simulink model "pll"  (Simulink 9.2)
settings: Solver=ode45  StartTime=0.0  StopTime=40  MaxStep=0.0001  RelTol=1e-3  EnableMultiTasking=on
libraries: simulink x2
settings Model: Creator=buddyugwumba1  LastModifiedBy=buddyugwumba1
settings OptimizationCC: InitFltsAndDblsToZero=on
settings DebuggingCC: SaveWithParameterizedLinksMsg=none  SignalResolutionControl=TryResolveAllWithWarning  SolverPrmCheckMsg=warning  MultiTaskDSMMsg=warning  MultiTaskCondExecSysMsg=none  FcnCallInpInsideContextMsg=error  StateNameClashWarn=none
settings SFSimCC: SimUseLocalCustomCode=on
settings RTWCC: RTWUseLocalCustomCode=on
settings GRTTargetCC: TargetFcnLib=ansi_tfl_tmw.mat  GeneratePreprocessorConditionals=Use local settings
settings ConfigComp: CovExternalEMLEnable=on

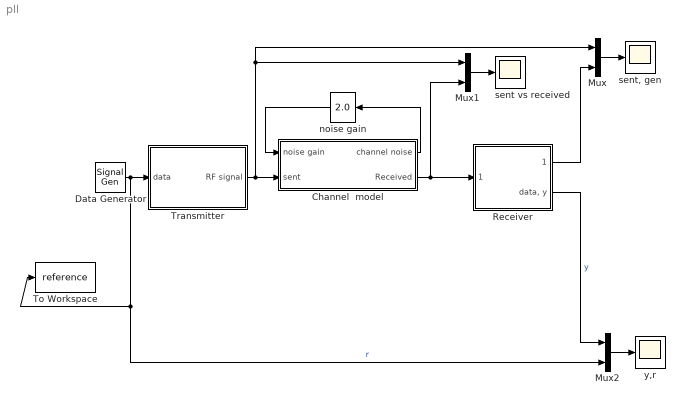
== system pll ==
  Channel  model : Subsystem
  Data Generator : SignalGenerator  WaveForm=square  Amplitude=2  Frequency=0.05
  Mux : Mux  Inputs=2
  Mux1 : Mux  Inputs=2
  Mux2 : Mux  Inputs=2
  Receiver : Subsystem
  To Workspace : ToWorkspace  VariableName=reference  SaveFormat=Structure With Time  SampleTime=-1
  Transmitter : Subsystem
  noise gain : simulink/Math Operations/Slider Gain  gain=2.0  low=0  high=2
  sent vs received : Scope
  "sent, gen" : Scope
  y,r : Scope
  wires:
  Mux/1 -> "sent, gen"/1
  Receiver/1(rep. sin) -> Mux/2
  Transmitter/1(RF signal) -> Channel  model/2(sent), Mux/1, Mux1/1
  Channel  model/2(Received) -> Receiver/1(rcvd. sig), Mux1/2
  Mux1/1 -> sent vs received/1
  Mux2/1 -> y,r/1
  Data Generator/1 -> To Workspace/1, Mux2/2, Transmitter/1(data)  "r"
  noise gain/1 -> Channel  model/1(noise gain)
  Channel  model/1(channel noise) -> noise gain/1
  Receiver/2("data, y") -> Mux2/1  "y"

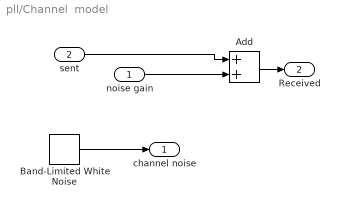
== system pll/Channel  model ==
  noise gain : Inport
  sent : Inport  Port=2
  Add : Sum
  Band-Limited White Noise : simulink/Sources/Band-Limited White Noise  Cov=[0.001]  Ts=0.0001  seed=[23341]
  channel noise : Outport
  Received : Outport  Port=2
  wires:
  sent/1 -> Add/1
  Add/1 -> Received/1
  Band-Limited White Noise/1 -> channel noise/1
  noise gain/1 -> Add/2

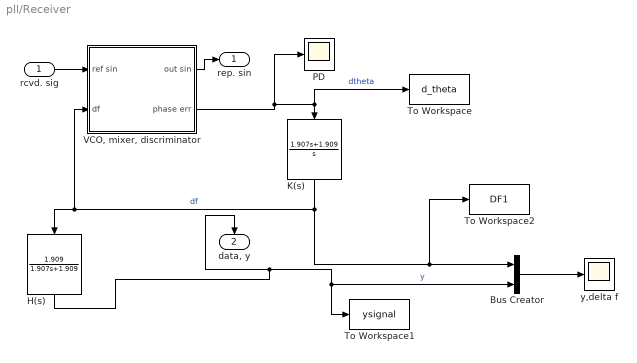
== system pll/Receiver ==
  rcvd. sig : Inport
  Bus Creator : BusCreator  Inputs=2
  H(s) : TransferFcn  Numerator=[1.909]  Denominator=[1.907 1.909]
  K(s) : TransferFcn  Numerator=[1.907 1.909]  Denominator=[1 0]
  PD : Scope
  To Workspace : ToWorkspace  VariableName=d_theta  SaveFormat=Timeseries  SampleTime=-1
  To Workspace1 : ToWorkspace  VariableName=ysignal  SaveFormat=Structure With Time  SampleTime=-1
  To Workspace2 : ToWorkspace  VariableName=DF1  SaveFormat=Structure With Time  SampleTime=-1
  "VCO, mixer, discriminator" : Subsystem
  y,delta f : Scope
  rep. sin : Outport
  "data, y" : Outport  Port=2
  wires:
  K(s)/1 -> To Workspace2/1, Bus Creator/1, H(s)/1, "VCO, mixer, discriminator"/2(df)  "df"
  "VCO, mixer, discriminator"/2(phase err) -> To Workspace/1, K(s)/1, PD/1  "dtheta"
  rcvd. sig/1 -> "VCO, mixer, discriminator"/1(ref sin)
  "VCO, mixer, discriminator"/1(out sin) -> rep. sin/1
  H(s)/1 -> Bus Creator/2, To Workspace1/1, "data, y"/1  "y"
  Bus Creator/1 -> y,delta f/1

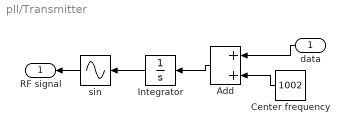
== system pll/Transmitter ==
  data : Inport
  Add : Sum
  Center frequency : Constant  Value=1002
  Integrator : Integrator  InitialCondition=pi/2
  sin : Sin  TimeSource=Use external signal  Frequency=2*pi  SampleTime=0
  RF signal : Outport
  wires:
  Integrator/1 -> sin/1
  Add/1 -> Integrator/1
  Center frequency/1 -> Add/2
  data/1 -> Add/1
  sin/1 -> RF signal/1

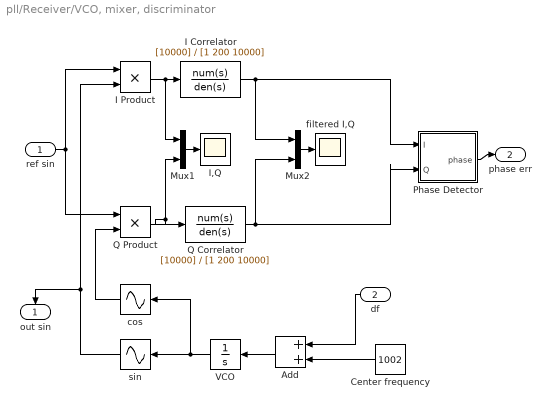
== system pll/Receiver/VCO, mixer, discriminator ==
  ref sin : Inport
  df : Inport  Port=2
  Add : Sum
  Center frequency : Constant  Value=1002
  I Correlator : TransferFcn  Numerator=[10000]  Denominator=[1 200 10000]
  I Product : Product  RndMeth=Zero
  I,Q : Scope
  Mux1 : Mux  Inputs=2
  Mux2 : Mux  Inputs=2
  Phase Detector : Subsystem
  Q Correlator : TransferFcn  Numerator=[10000]  Denominator=[1 200 10000]
  Q Product : Product  RndMeth=Zero
  VCO : Integrator  InitialCondition=pi/2
  cos : Sin  TimeSource=Use external signal  Frequency=2*pi  Phase=pi/2  SampleTime=0
  filtered I,Q : Scope
  sin : Sin  TimeSource=Use external signal  Frequency=2*pi  SampleTime=0
  out sin : Outport
  phase err : Outport  Port=2
  wires:
  VCO/1 -> sin/1, cos/1
  sin/1 -> I Product/2, out sin/1
  I Product/1 -> Mux1/1, I Correlator/1
  Add/1 -> VCO/1
  Center frequency/1 -> Add/2
  Q Product/1 -> Mux1/2, Q Correlator/1
  cos/1 -> Q Product/2
  Mux1/1 -> I,Q/1
  I Correlator/1 -> Mux2/1, Phase Detector/1(I)
  Q Correlator/1 -> Mux2/2, Phase Detector/2(Q)
  Mux2/1 -> filtered I,Q/1
  ref sin/1 -> I Product/1, Q Product/1
  df/1 -> Add/1
  Phase Detector/1(phase) -> phase err/1

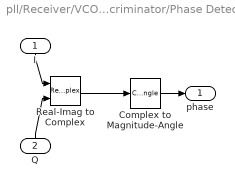
== system pll/Receiver/VCO, mixer, discriminator/Phase Detector ==
  I : Inport
  Q : Inport  Port=2
  Complex to Magnitude-Angle : ComplexToMagnitudeAngle  Output=Angle
  Real-Imag to Complex : RealImagToComplex
  phase : Outport
  wires:
  Real-Imag to Complex/1 -> Complex to Magnitude-Angle/1
  I/1 -> Real-Imag to Complex/1
  Q/1 -> Real-Imag to Complex/2
  Complex to Magnitude-Angle/1 -> phase/1
